simulink model "ExampleBlindSpot"  (Simulink 9.2)
settings: Solver=FixedStepDiscrete  StartTime=0.0  StopTime=Inf  FixedStep=0.001  RelTol=1e-3  EnableMultiTasking=on
libraries: simulink x30, rFproPhysicsLib x6, simulink_extras x3
settings Model: Creator=SeanK  LastModifiedBy=SeanKavanagh
settings DataIOCC: SignalLoggingSaveFormat=Dataset
settings DebuggingCC: SolverPrmCheckMsg=warning  FcnCallInpInsideContextMsg=error  StateNameClashWarn=none
settings RTWCC: SystemTargetFile=rfpro.tlc  MakeCommand="make_rtw OPTS=\"-DRUN_PHYSICS\""  TemplateMakefile=rfpro.tmf  Description=rFpro Target (Run Physics)  TargetLang=C++
settings STFCustomTargetCC: ModelReferenceCompliant=off  GeneratePreprocessorConditionals=Disable all  CombineOutputUpdateFcns=on  MatFileLogging=on  CPPClassGenCompliant=on  GRTInterface=off  SystemTargetFile=rfpro.tlc
settings GRTTargetCC: ModelReferenceCompliant=off  ParMdlRefBuildCompliant=off  CompOptLevelCompliant=off  ConcurrentExecutionCompliant=off  CombineOutputUpdateFcns=on  GRTInterface=off  UseToolchainInfoCompliant=off

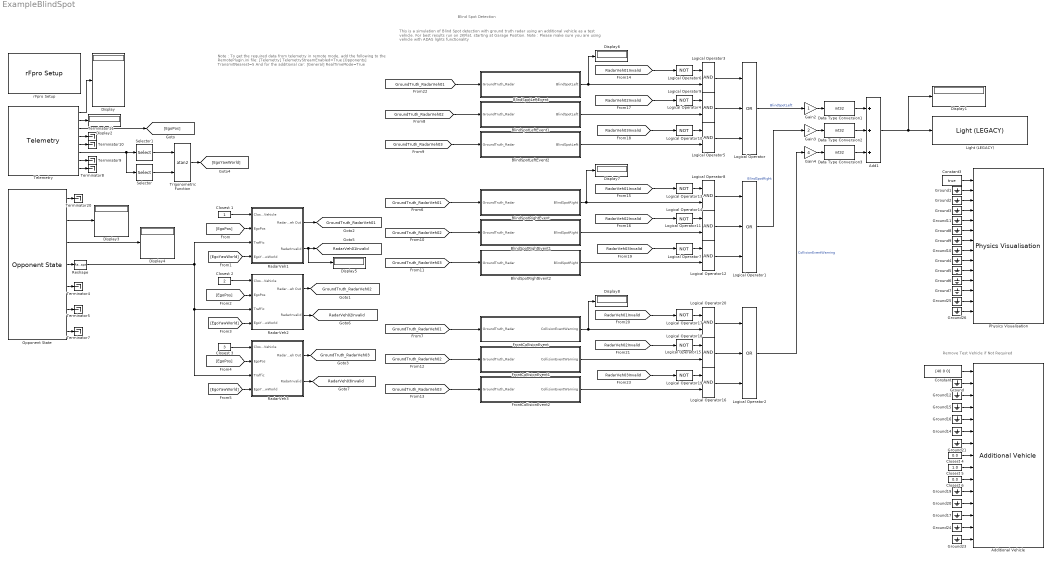
== system ExampleBlindSpot ==
  note: This is a simulation of Blind Spot detection with ground truth radar using an additional vehicle as a test vehicle.
      | For best results run on 2KFlat, starting at Garage Position.
      | Note : Please make sure you are using vehicle with ADAS lights functionality
  note: Remove Test Vehicle if Not Required
  note: Blind Spot Detection
  note: Note : To get the required data from telemetry in remote mode,
      | add the following to the RemotePlugin.ini file:
      |
      | [Telemetry]
      | TelemetryStreamEnabled=True
      |
      | [Opponents]
      | TransmitNearest=5
      |
      | And for the additional car:
      |
      | [General]
      | RealTimeMode=True
  Add1 : Sum  Inputs=+++
  Additional Vehicle : rFproPhysicsLib/Additional Vehicle  VEH_FILE='Hatchback_AWD_Red'  DRIVER_NAME=''  UPGRADE_PACK=0  SKIN=''  HELMET=''  COLLIDABLE=off  TRANSPARENT_PROXIMITY=0  MANUAL_TRANSPARENCY=0  HEIGHT_VALID=off  ORI_VALID=off  HEADING_VALID=off  VEL_VALID=off  ROT_VALID=off  GEAR_VALID=off  RPM_VALID=off  INPUTS_VALID=on  BRAKE_LIGHT_VALID=off  HEADLIGHT_VALID=off  WHEEL_ROTATIONS_VALID=off  WHEEL_BRAKE_TEMPS_VALID=off  WHEEL_HEIGHTS_VALID=off  period=-1  offset=0  useReverseByteOrder=on  rFpro__platform=Remote Model - Default
  BlindSpotLeftEvent : Subsystem
  BlindSpotLeftEvent1 : Subsystem
  BlindSpotLeftEvent2 : Subsystem
  BlindSpotRightEvent : Subsystem
  BlindSpotRightEvent1 : Subsystem
  BlindSpotRightEvent2 : Subsystem
  Closest 1 : Constant
  Closest 2 : Constant  Value=2
  Closest 3 : Constant  Value=3
  Closest 4 : Constant  Value=0.0
  Closest 5 : Constant  Value=1.0
  Closest 6 : Constant  Value=0.0
  Constant : Constant  Value=[40 0 0]
  Constant3 : Constant  Value=true
  Data Type Conversion1 : DataTypeConversion  OutDataTypeStr=int32
  Data Type Conversion2 : DataTypeConversion  OutDataTypeStr=int32
  Data Type Conversion3 : DataTypeConversion  OutDataTypeStr=int32
  Display{,1..8} (9 alike) : Display
  FrontCollisionEvent : Subsystem
  FrontCollisionEvent1 : Subsystem
  FrontCollisionEvent2 : Subsystem
  Gain2 : Gain
  Gain3 : Gain  Gain=2
  Gain4 : Gain  Gain=4
  Ground{,1..12,14..17,19..21,23..26} (24 alike) : Ground
  Light (LEGACY) : rFproPhysicsLib/Legacy Blocks/Light (LEGACY)  light_name='LIGHTSADAS'  exact_match=off  on_vehicle=on  useReverseByteOrder=off  rFpro__platform=Remote Model - Default
  Logical Operator : Logic  Operator=OR  Inputs=3  AllPortsSameDT=off  OutDataTypeStr=boolean
  Logical Operator1 : Logic  Operator=OR  Inputs=3  AllPortsSameDT=off  OutDataTypeStr=boolean
  Logical Operator{6..7,9..10,13..14,17..19} (9 alike) : Logic  Operator=NOT  AllPortsSameDT=off  OutDataTypeStr=boolean
  Logical Operator{3..5,8,11..12,15..16,20} (9 alike) : Logic  AllPortsSameDT=off  OutDataTypeStr=boolean
  Logical Operator2 : Logic  Operator=OR  Inputs=3  AllPortsSameDT=off  OutDataTypeStr=boolean
  Opponent State : rFproPhysicsLib/Opponent State  max_SL_opponents=3  flattenOutput=on
  Physics Visualisation : rFproPhysicsLib/Physics Visualisation  PAR_SKIP_INTERNAL_PHYSICS=off  PAR_ACCEL_VALID=off  PAR_ROT_ACCEL_VALID=off  PAR_GEAR_VALID=off  PAR_RPM_VALID=off  PAR_INPUTS_VALID=on  PAR_STEER_TORQUE_VALID=off  PAR_HEADLIGHTS_ON_VALID=off  PAR_WHEEL_POS_VALID=off  PAR_WHEEL_ORI_VALID=off  PAR_TYRE_PARAMS_VALID=off  PAR_WHEEL_ROTATION_VALID=off  PAR_WHEEL_BRAKE_TEMP_VALID=off  PAR_WHEEL_TREAD_TEMP_VALID=off  PAR_WHEEL_AIR_TEMP_VALID=off  period=-1  offset=0  useReverseByteOrder=on  rFpro__platform=Remote Model - Default
  RadarVeh1 : Subsystem
  RadarVeh2 : Subsystem
  RadarVeh3 : Subsystem
  Reshape : Reshape  OutputDimensionality=Customize  OutputDimensions=[3,3]
  Selector : Selector  NumberOfDimensions=2  InputPortWidth=3  IndexOptions=Index vector (dialog),Index vector (dialog)  Indices=1,1  OutputSizes=1,1
  Selector1 : Selector  NumberOfDimensions=2  InputPortWidth=3  IndexOptions=Index vector (dialog),Index vector (dialog)  Indices=1,2  OutputSizes=1,1
  Telemetry : rFproPhysicsLib/Telemetry
  Terminator{4..5,7..11,20} (8 alike) : Terminator
  Trigonometric Function : Trigonometry  Operator=atan2
  rFpro Setup : rFproPhysicsLib/rFpro Setup  platform=Remote Model - Default  stopOnSessionEnd=on  usePseudoRealtime=on  syncToRF=on  useReverseByteOrder=off  useRfTime=on  minIterations=4  maxIterations=1000  ipReceiveAddress='127.0.0.1'  ipReceivePort=11054  receiveSampleTime=-1  ipTransmitAddress='127.0.0.1'  ipTransmitPort=11052  transmitSampleTime=0.001  pluginType=RUN_PHYSICS  sysTarget=xpctarget.tlc  templateMakeFile=xpc_default_tmf  makeCommand=make_rtw  buildDesc=xPC target
  tag scope: GroundTruth_RadarVeh01=global, GroundTruth_RadarVeh02=global, GroundTruth_RadarVeh03=global, RadarVeh01Invalid=global, RadarVeh02Invalid=global, RadarVeh03Invalid=global
  wires:
  Constant3/1 -> Physics Visualisation/1
  Ground8/1 -> Physics Visualisation/6
  Ground9/1 -> Physics Visualisation/7
  Ground10/1 -> Physics Visualisation/8
  Ground11/1 -> Physics Visualisation/5
  Ground1/1 -> Physics Visualisation/2
  Ground2/1 -> Physics Visualisation/3
  Ground3/1 -> Physics Visualisation/4
  Opponent State/2 -> Display3/1
  Opponent State/5 -> Terminator4/1
  Opponent State/6 -> Terminator5/1
  Closest 1/1 -> RadarVeh1/1(Closest Vehicle)
  Telemetry/3 -> [EgoPos]
  [EgoYawWorld] -> RadarVeh1/4(EgoYawWorld)
  [EgoPos] -> RadarVeh1/2(EgoPos)
  [EgoPos] -> RadarVeh2/2(EgoPos)
  [EgoYawWorld] -> RadarVeh2/4(EgoYawWorld)
  Closest 2/1 -> RadarVeh2/1(Closest Vehicle)
  Closest 3/1 -> RadarVeh3/1(Closest Vehicle)
  [EgoYawWorld] -> RadarVeh3/4(EgoYawWorld)
  [EgoPos] -> RadarVeh3/2(EgoPos)
  RadarVeh1/1(RadarVeh Out) -> [GroundTruth_RadarVeh01]
  RadarVeh2/1(RadarVeh Out) -> [GroundTruth_RadarVeh02]
  RadarVeh3/1(RadarVeh Out) -> [GroundTruth_RadarVeh03]
  Logical Operator2/1 -> Gain4/1  "CollisionEventWarning"
  Logical Operator/1 -> Gain2/1  "BlindSpotLeft"
  Logical Operator1/1 -> Gain3/1  "BlindSpotRight"
  [GroundTruth_RadarVeh03] -> FrontCollisionEvent2/1(GroundTruth_Radar)
  [GroundTruth_RadarVeh02] -> FrontCollisionEvent1/1(GroundTruth_Radar)
  [GroundTruth_RadarVeh03] -> BlindSpotRightEvent2/1(GroundTruth_Radar)
  [GroundTruth_RadarVeh02] -> BlindSpotRightEvent1/1(GroundTruth_Radar)
  BlindSpotLeftEvent2/1(BlindSpotLeft) -> Logical Operator5/2
  [GroundTruth_RadarVeh03] -> BlindSpotLeftEvent2/1(GroundTruth_Radar)
  [GroundTruth_RadarVeh02] -> BlindSpotLeftEvent1/1(GroundTruth_Radar)
  BlindSpotLeftEvent1/1(BlindSpotLeft) -> Logical Operator4/2
  [GroundTruth_RadarVeh01] -> FrontCollisionEvent/1(GroundTruth_Radar)
  [GroundTruth_RadarVeh01] -> BlindSpotRightEvent/1(GroundTruth_Radar)
  BlindSpotLeftEvent/1(BlindSpotLeft) -> Display6/1, Logical Operator3/2
  [GroundTruth_RadarVeh01] -> BlindSpotLeftEvent/1(GroundTruth_Radar)
  Gain4/1 -> Data Type Conversion3/1
  Add1/1 -> Light (LEGACY)/1, Display1/1
  Gain3/1 -> Data Type Conversion2/1
  Data Type Conversion1/1 -> Add1/1
  Data Type Conversion3/1 -> Add1/3
  Data Type Conversion2/1 -> Add1/2
  Gain2/1 -> Data Type Conversion1/1
  Trigonometric Function/1 -> [EgoYawWorld]
  Constant/1 -> Additional Vehicle/1
  Ground/1 -> Additional Vehicle/2
  Ground19/1 -> Additional Vehicle/11
  Ground16/1 -> Additional Vehicle/5
  Ground15/1 -> Additional Vehicle/4
  Ground12/1 -> Additional Vehicle/3
  Ground20/1 -> Additional Vehicle/12
  Ground17/1 -> Additional Vehicle/13
  Ground14/1 -> Additional Vehicle/6
  Ground21/1 -> Additional Vehicle/7
  Ground24/1 -> Additional Vehicle/14
  Ground23/1 -> Additional Vehicle/15
  Telemetry/6 -> Selector/1, Selector1/1
  Selector1/1 -> Trigonometric Function/1
  Selector/1 -> Trigonometric Function/2
  RadarVeh1/2(RadarInvalid) -> Display5/1, [RadarVeh01Invalid]
  RadarVeh2/2(RadarInvalid) -> [RadarVeh02Invalid]
  RadarVeh3/2(RadarInvalid) -> [RadarVeh03Invalid]
  [RadarVeh01Invalid] -> Logical Operator6/1
  Logical Operator6/1 -> Logical Operator3/1
  Logical Operator3/1 -> Logical Operator/1
  Logical Operator4/1 -> Logical Operator/2
  Logical Operator5/1 -> Logical Operator/3
  Logical Operator9/1 -> Logical Operator4/1
  [RadarVeh02Invalid] -> Logical Operator9/1
  [RadarVeh03Invalid] -> Logical Operator10/1
  Logical Operator10/1 -> Logical Operator5/1
  Logical Operator7/1 -> Logical Operator12/1
  [RadarVeh03Invalid] -> Logical Operator7/1
  [RadarVeh02Invalid] -> Logical Operator14/1
  Logical Operator14/1 -> Logical Operator11/1
  Logical Operator12/1 -> Logical Operator1/3
  Logical Operator11/1 -> Logical Operator1/2
  Logical Operator8/1 -> Logical Operator1/1
  Logical Operator13/1 -> Logical Operator8/1
  [RadarVeh01Invalid] -> Logical Operator13/1
  BlindSpotRightEvent/1(BlindSpotRight) -> Display7/1, Logical Operator8/2
  BlindSpotRightEvent1/1(BlindSpotRight) -> Logical Operator11/2
  BlindSpotRightEvent2/1(BlindSpotRight) -> Logical Operator12/2
  FrontCollisionEvent2/1(CollisionEventWarning) -> Logical Operator16/2
  FrontCollisionEvent1/1(CollisionEventWarning) -> Logical Operator15/2
  FrontCollisionEvent/1(CollisionEventWarning) -> Display8/1, Logical Operator20/2
  [RadarVeh01Invalid] -> Logical Operator17/1
  Logical Operator17/1 -> Logical Operator20/1
  Logical Operator20/1 -> Logical Operator2/1
  Logical Operator15/1 -> Logical Operator2/2
  Logical Operator16/1 -> Logical Operator2/3
  Logical Operator18/1 -> Logical Operator15/1
  [RadarVeh02Invalid] -> Logical Operator18/1
  [RadarVeh03Invalid] -> Logical Operator19/1
  Logical Operator19/1 -> Logical Operator16/1
  Opponent State/1 -> Terminator20/1
  Ground4/1 -> Physics Visualisation/9
  Ground5/1 -> Physics Visualisation/10
  Ground6/1 -> Physics Visualisation/11
  Ground7/1 -> Physics Visualisation/12
  Ground26/1 -> Physics Visualisation/14
  Ground25/1 -> Physics Visualisation/13
  Opponent State/7 -> Terminator7/1
  Opponent State/4 -> Reshape/1
  Telemetry/1 -> Display/1
  Telemetry/2 -> Display2/1
  Telemetry/4 -> Terminator11/1
  Telemetry/5 -> Terminator10/1
  Telemetry/7 -> Terminator9/1
  Telemetry/8 -> Terminator8/1
  Opponent State/3 -> Display4/1
  Reshape/1 -> RadarVeh1/3(Traffic), RadarVeh3/3(Traffic), RadarVeh2/3(Traffic)
  Closest 4/1 -> Additional Vehicle/8
  Closest 5/1 -> Additional Vehicle/9
  Closest 6/1 -> Additional Vehicle/10

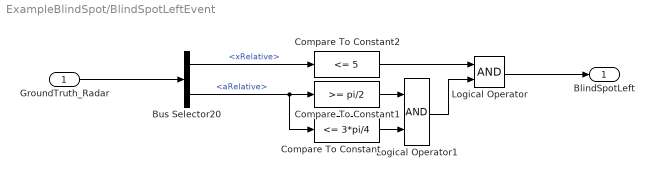
== system ExampleBlindSpot/BlindSpotLeftEvent ==
  GroundTruth_Radar : Inport
  Bus Selector20 : BusSelector  OutputSignals=xRelative,aRelative
  Compare To Constant : simulink/Logic and Bit Operations/Compare To Constant  relop=<=  const=3*pi/4  OutDataTypeStr=boolean
  Compare To Constant1 : simulink/Logic and Bit Operations/Compare To Constant  relop=>=  const=pi/2  OutDataTypeStr=boolean
  Compare To Constant2 : simulink/Logic and Bit Operations/Compare To Constant  relop=<=  const=5  OutDataTypeStr=boolean
  Logical Operator : Logic  AllPortsSameDT=off  OutDataTypeStr=boolean
  Logical Operator1 : Logic  AllPortsSameDT=off  OutDataTypeStr=boolean
  BlindSpotLeft : Outport
  wires:
  Logical Operator/1 -> BlindSpotLeft/1
  Compare To Constant2/1 -> Logical Operator/1
  Logical Operator1/1 -> Logical Operator/2
  Bus Selector20/1 -> Compare To Constant2/1  "<xRelative>"
  GroundTruth_Radar/1 -> Bus Selector20/1
  Compare To Constant1/1 -> Logical Operator1/1
  Bus Selector20/2 -> Compare To Constant/1, Compare To Constant1/1  "<aRelative>"
  Compare To Constant/1 -> Logical Operator1/2

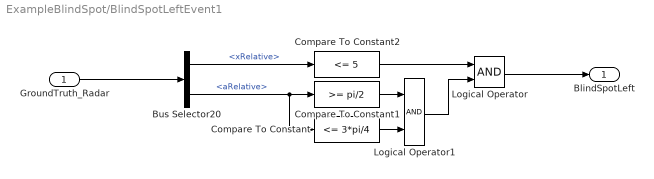
== system ExampleBlindSpot/BlindSpotLeftEvent1 ==
  GroundTruth_Radar : Inport
  Bus Selector20 : BusSelector  OutputSignals=xRelative,aRelative
  Compare To Constant : simulink/Logic and Bit Operations/Compare To Constant  relop=<=  const=3*pi/4  OutDataTypeStr=boolean
  Compare To Constant1 : simulink/Logic and Bit Operations/Compare To Constant  relop=>=  const=pi/2  OutDataTypeStr=boolean
  Compare To Constant2 : simulink/Logic and Bit Operations/Compare To Constant  relop=<=  const=5  OutDataTypeStr=boolean
  Logical Operator : Logic  AllPortsSameDT=off  OutDataTypeStr=boolean
  Logical Operator1 : Logic  AllPortsSameDT=off  OutDataTypeStr=boolean
  BlindSpotLeft : Outport
  wires:
  Logical Operator/1 -> BlindSpotLeft/1
  Compare To Constant2/1 -> Logical Operator/1
  Logical Operator1/1 -> Logical Operator/2
  Bus Selector20/1 -> Compare To Constant2/1  "<xRelative>"
  GroundTruth_Radar/1 -> Bus Selector20/1
  Compare To Constant1/1 -> Logical Operator1/1
  Bus Selector20/2 -> Compare To Constant/1, Compare To Constant1/1  "<aRelative>"
  Compare To Constant/1 -> Logical Operator1/2

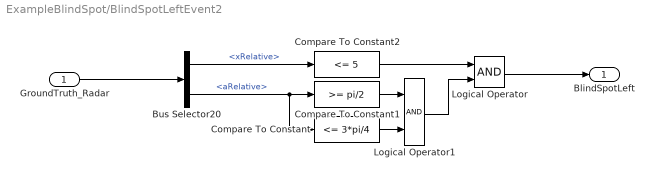
== system ExampleBlindSpot/BlindSpotLeftEvent2 ==
  GroundTruth_Radar : Inport
  Bus Selector20 : BusSelector  OutputSignals=xRelative,aRelative
  Compare To Constant : simulink/Logic and Bit Operations/Compare To Constant  relop=<=  const=3*pi/4  OutDataTypeStr=boolean
  Compare To Constant1 : simulink/Logic and Bit Operations/Compare To Constant  relop=>=  const=pi/2  OutDataTypeStr=boolean
  Compare To Constant2 : simulink/Logic and Bit Operations/Compare To Constant  relop=<=  const=5  OutDataTypeStr=boolean
  Logical Operator : Logic  AllPortsSameDT=off  OutDataTypeStr=boolean
  Logical Operator1 : Logic  AllPortsSameDT=off  OutDataTypeStr=boolean
  BlindSpotLeft : Outport
  wires:
  Logical Operator/1 -> BlindSpotLeft/1
  Compare To Constant2/1 -> Logical Operator/1
  Logical Operator1/1 -> Logical Operator/2
  Bus Selector20/1 -> Compare To Constant2/1  "<xRelative>"
  GroundTruth_Radar/1 -> Bus Selector20/1
  Compare To Constant1/1 -> Logical Operator1/1
  Bus Selector20/2 -> Compare To Constant/1, Compare To Constant1/1  "<aRelative>"
  Compare To Constant/1 -> Logical Operator1/2

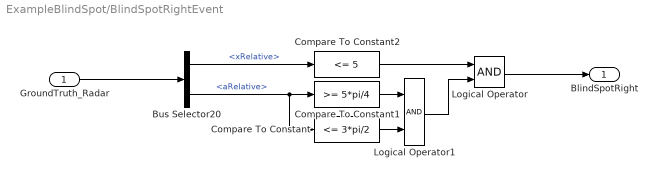
== system ExampleBlindSpot/BlindSpotRightEvent ==
  GroundTruth_Radar : Inport
  Bus Selector20 : BusSelector  OutputSignals=xRelative,aRelative
  Compare To Constant : simulink/Logic and Bit Operations/Compare To Constant  relop=<=  const=3*pi/2  OutDataTypeStr=boolean
  Compare To Constant1 : simulink/Logic and Bit Operations/Compare To Constant  relop=>=  const=5*pi/4  OutDataTypeStr=boolean
  Compare To Constant2 : simulink/Logic and Bit Operations/Compare To Constant  relop=<=  const=5  OutDataTypeStr=boolean
  Logical Operator : Logic  AllPortsSameDT=off  OutDataTypeStr=boolean
  Logical Operator1 : Logic  AllPortsSameDT=off  OutDataTypeStr=boolean
  BlindSpotRight : Outport
  wires:
  Compare To Constant/1 -> Logical Operator1/2
  Bus Selector20/2 -> Compare To Constant/1, Compare To Constant1/1  "<aRelative>"
  Compare To Constant1/1 -> Logical Operator1/1
  GroundTruth_Radar/1 -> Bus Selector20/1
  Bus Selector20/1 -> Compare To Constant2/1  "<xRelative>"
  Logical Operator1/1 -> Logical Operator/2
  Compare To Constant2/1 -> Logical Operator/1
  Logical Operator/1 -> BlindSpotRight/1

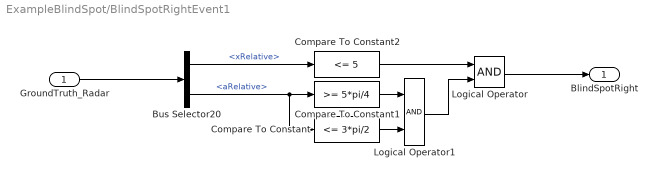
== system ExampleBlindSpot/BlindSpotRightEvent1 ==
  GroundTruth_Radar : Inport
  Bus Selector20 : BusSelector  OutputSignals=xRelative,aRelative
  Compare To Constant : simulink/Logic and Bit Operations/Compare To Constant  relop=<=  const=3*pi/2  OutDataTypeStr=boolean
  Compare To Constant1 : simulink/Logic and Bit Operations/Compare To Constant  relop=>=  const=5*pi/4  OutDataTypeStr=boolean
  Compare To Constant2 : simulink/Logic and Bit Operations/Compare To Constant  relop=<=  const=5  OutDataTypeStr=boolean
  Logical Operator : Logic  AllPortsSameDT=off  OutDataTypeStr=boolean
  Logical Operator1 : Logic  AllPortsSameDT=off  OutDataTypeStr=boolean
  BlindSpotRight : Outport
  wires:
  Compare To Constant/1 -> Logical Operator1/2
  Bus Selector20/2 -> Compare To Constant/1, Compare To Constant1/1  "<aRelative>"
  Compare To Constant1/1 -> Logical Operator1/1
  GroundTruth_Radar/1 -> Bus Selector20/1
  Bus Selector20/1 -> Compare To Constant2/1  "<xRelative>"
  Logical Operator1/1 -> Logical Operator/2
  Compare To Constant2/1 -> Logical Operator/1
  Logical Operator/1 -> BlindSpotRight/1

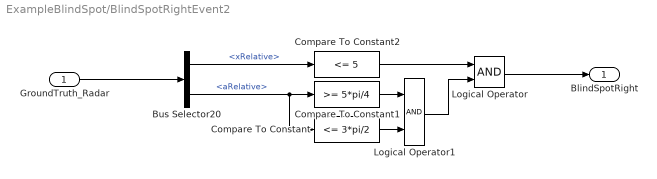
== system ExampleBlindSpot/BlindSpotRightEvent2 ==
  GroundTruth_Radar : Inport
  Bus Selector20 : BusSelector  OutputSignals=xRelative,aRelative
  Compare To Constant : simulink/Logic and Bit Operations/Compare To Constant  relop=<=  const=3*pi/2  OutDataTypeStr=boolean
  Compare To Constant1 : simulink/Logic and Bit Operations/Compare To Constant  relop=>=  const=5*pi/4  OutDataTypeStr=boolean
  Compare To Constant2 : simulink/Logic and Bit Operations/Compare To Constant  relop=<=  const=5  OutDataTypeStr=boolean
  Logical Operator : Logic  AllPortsSameDT=off  OutDataTypeStr=boolean
  Logical Operator1 : Logic  AllPortsSameDT=off  OutDataTypeStr=boolean
  BlindSpotRight : Outport
  wires:
  Compare To Constant/1 -> Logical Operator1/2
  Bus Selector20/2 -> Compare To Constant/1, Compare To Constant1/1  "<aRelative>"
  Compare To Constant1/1 -> Logical Operator1/1
  GroundTruth_Radar/1 -> Bus Selector20/1
  Bus Selector20/1 -> Compare To Constant2/1  "<xRelative>"
  Logical Operator1/1 -> Logical Operator/2
  Compare To Constant2/1 -> Logical Operator/1
  Logical Operator/1 -> BlindSpotRight/1

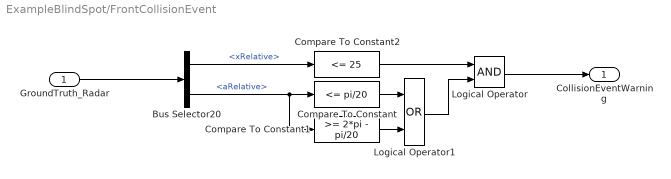
== system ExampleBlindSpot/FrontCollisionEvent ==
  GroundTruth_Radar : Inport
  Bus Selector20 : BusSelector  OutputSignals=xRelative,aRelative
  Compare To Constant : simulink/Logic and Bit Operations/Compare To Constant  relop=<=  const=pi/20  OutDataTypeStr=boolean
  Compare To Constant1 : simulink/Logic and Bit Operations/Compare To Constant  relop=>=  const=2*pi - pi/20  OutDataTypeStr=boolean
  Compare To Constant2 : simulink/Logic and Bit Operations/Compare To Constant  relop=<=  const=25  OutDataTypeStr=boolean
  Logical Operator : Logic  AllPortsSameDT=off  OutDataTypeStr=boolean
  Logical Operator1 : Logic  Operator=OR  AllPortsSameDT=off  OutDataTypeStr=boolean
  CollisionEventWarning : Outport
  wires:
  Compare To Constant/1 -> Logical Operator1/1
  Bus Selector20/2 -> Compare To Constant1/1, Compare To Constant/1  "<aRelative>"
  Compare To Constant1/1 -> Logical Operator1/2
  GroundTruth_Radar/1 -> Bus Selector20/1
  Bus Selector20/1 -> Compare To Constant2/1  "<xRelative>"
  Logical Operator1/1 -> Logical Operator/2
  Compare To Constant2/1 -> Logical Operator/1
  Logical Operator/1 -> CollisionEventWarning/1

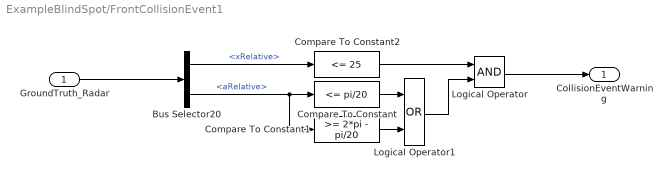
== system ExampleBlindSpot/FrontCollisionEvent1 ==
  GroundTruth_Radar : Inport
  Bus Selector20 : BusSelector  OutputSignals=xRelative,aRelative
  Compare To Constant : simulink/Logic and Bit Operations/Compare To Constant  relop=<=  const=pi/20  OutDataTypeStr=boolean
  Compare To Constant1 : simulink/Logic and Bit Operations/Compare To Constant  relop=>=  const=2*pi - pi/20  OutDataTypeStr=boolean
  Compare To Constant2 : simulink/Logic and Bit Operations/Compare To Constant  relop=<=  const=25  OutDataTypeStr=boolean
  Logical Operator : Logic  AllPortsSameDT=off  OutDataTypeStr=boolean
  Logical Operator1 : Logic  Operator=OR  AllPortsSameDT=off  OutDataTypeStr=boolean
  CollisionEventWarning : Outport
  wires:
  Compare To Constant/1 -> Logical Operator1/1
  Bus Selector20/2 -> Compare To Constant1/1, Compare To Constant/1  "<aRelative>"
  Compare To Constant1/1 -> Logical Operator1/2
  GroundTruth_Radar/1 -> Bus Selector20/1
  Bus Selector20/1 -> Compare To Constant2/1  "<xRelative>"
  Logical Operator1/1 -> Logical Operator/2
  Compare To Constant2/1 -> Logical Operator/1
  Logical Operator/1 -> CollisionEventWarning/1

== system ExampleBlindSpot/FrontCollisionEvent2 ==
  GroundTruth_Radar : Inport
  Bus Selector20 : BusSelector  OutputSignals=xRelative,aRelative
  Compare To Constant : simulink/Logic and Bit Operations/Compare To Constant  relop=<=  const=pi/20  OutDataTypeStr=boolean
  Compare To Constant1 : simulink/Logic and Bit Operations/Compare To Constant  relop=>=  const=2*pi - pi/20  OutDataTypeStr=boolean
  Compare To Constant2 : simulink/Logic and Bit Operations/Compare To Constant  relop=<=  const=25  OutDataTypeStr=boolean
  Logical Operator : Logic  AllPortsSameDT=off  OutDataTypeStr=boolean
  Logical Operator1 : Logic  Operator=OR  AllPortsSameDT=off  OutDataTypeStr=boolean
  CollisionEventWarning : Outport
  wires:
  Compare To Constant/1 -> Logical Operator1/1
  Bus Selector20/2 -> Compare To Constant1/1, Compare To Constant/1  "<aRelative>"
  Compare To Constant1/1 -> Logical Operator1/2
  GroundTruth_Radar/1 -> Bus Selector20/1
  Bus Selector20/1 -> Compare To Constant2/1  "<xRelative>"
  Logical Operator1/1 -> Logical Operator/2
  Compare To Constant2/1 -> Logical Operator/1
  Logical Operator/1 -> CollisionEventWarning/1

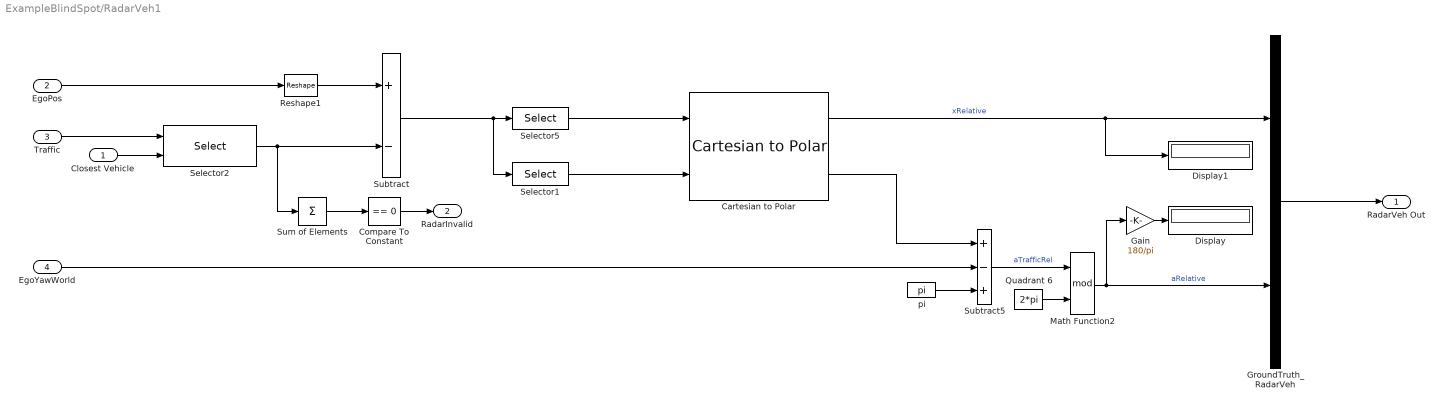
== system ExampleBlindSpot/RadarVeh1 ==
  Closest Vehicle : Inport
  EgoPos : Inport  Port=2
  Traffic : Inport  Port=3
  EgoYawWorld : Inport  Port=4
  Cartesian to Polar : simulink_extras/Transformations/Cartesian to Polar
      settings: SourceProductName=Simulink
  Compare To Constant : simulink/Logic and Bit Operations/Compare To Constant  relop===  const=0  OutDataTypeStr=boolean
  Display : Display
  Display1 : Display
  Gain : Gain  Gain=180/pi
  GroundTruth_RadarVeh : BusCreator  Inputs=2
  Math Function2 : Math  Operator=mod  SaturateOnIntegerOverflow=on
  Quadrant 6 : Constant  Value=2*pi
  Reshape1 : Reshape  OutputDimensionality=Column vector (2-D)
  Selector1 : Selector  InputPortWidth=3  IndexOptions=Index vector (dialog)  Indices=2  OutputSizes=1
  Selector2 : Selector  NumberOfDimensions=2  InputPortWidth=3  IndexOptions=Select all,Index vector (port)  Indices=[1 2 3],[1 2 3]  OutputSizes=1,1
  Selector5 : Selector  InputPortWidth=3  IndexOptions=Index vector (dialog)  Indices=1  OutputSizes=1
  Subtract : Sum  Inputs=+-
  Subtract5 : Sum  Inputs=+-+
  Sum of Elements : Sum  Inputs=+
  pi : Constant  Value=pi
  RadarVeh Out : Outport
  RadarInvalid : Outport  Port=2
  wires:
  Math Function2/1 -> GroundTruth_RadarVeh/2, Gain/1  "aRelative"
  EgoYawWorld/1 -> Subtract5/2
  Cartesian to Polar/1 -> Display1/1, GroundTruth_RadarVeh/1  "xRelative"
  Reshape1/1 -> Subtract/1
  Closest Vehicle/1 -> Selector2/2
  EgoPos/1 -> Reshape1/1
  Traffic/1 -> Selector2/1
  Selector2/1 -> Sum of Elements/1, Subtract/2
  GroundTruth_RadarVeh/1 -> RadarVeh Out/1
  pi/1 -> Subtract5/3
  Quadrant 6/1 -> Math Function2/2
  Subtract5/1 -> Math Function2/1  "aTrafficRel"
  Cartesian to Polar/2 -> Subtract5/1
  Selector5/1 -> Cartesian to Polar/1
  Selector1/1 -> Cartesian to Polar/2
  Subtract/1 -> Selector1/1, Selector5/1
  Compare To Constant/1 -> RadarInvalid/1
  Sum of Elements/1 -> Compare To Constant/1
  Gain/1 -> Display/1

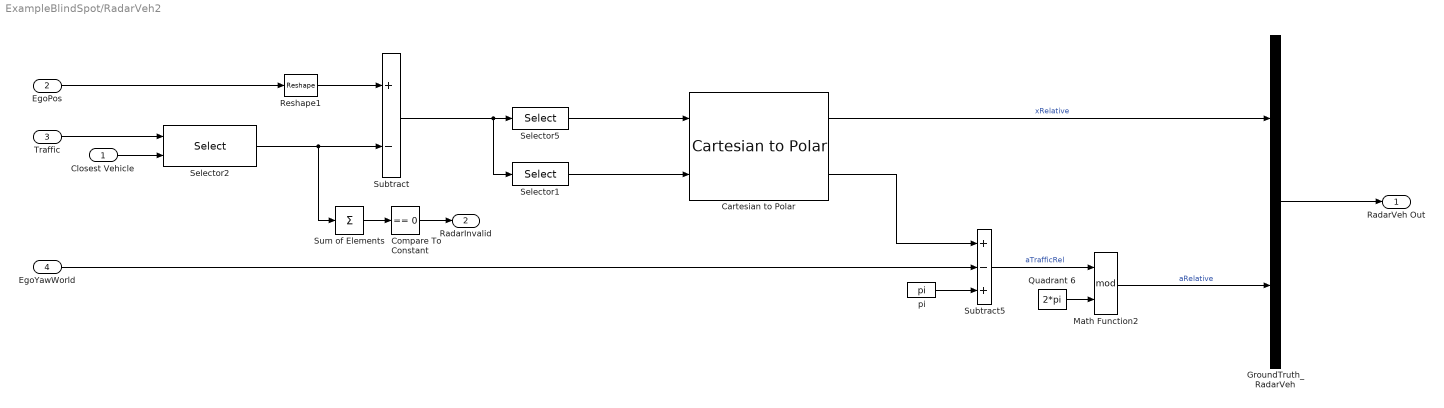
== system ExampleBlindSpot/RadarVeh2 ==
  Closest Vehicle : Inport
  EgoPos : Inport  Port=2
  Traffic : Inport  Port=3
  EgoYawWorld : Inport  Port=4
  Cartesian to Polar : simulink_extras/Transformations/Cartesian to Polar
      settings: SourceProductName=Simulink
  Compare To Constant : simulink/Logic and Bit Operations/Compare To Constant  relop===  const=0  OutDataTypeStr=boolean
  GroundTruth_RadarVeh : BusCreator  Inputs=2
  Math Function2 : Math  Operator=mod  SaturateOnIntegerOverflow=on
  Quadrant 6 : Constant  Value=2*pi
  Reshape1 : Reshape  OutputDimensionality=Column vector (2-D)
  Selector1 : Selector  InputPortWidth=3  IndexOptions=Index vector (dialog)  Indices=2  OutputSizes=1
  Selector2 : Selector  NumberOfDimensions=2  InputPortWidth=3  IndexOptions=Index vector (dialog),Index vector (port)  Indices=[1 2 3],[1 2 3]  OutputSizes=1,1
  Selector5 : Selector  InputPortWidth=3  IndexOptions=Index vector (dialog)  Indices=1  OutputSizes=1
  Subtract : Sum  Inputs=+-
  Subtract5 : Sum  Inputs=+-+
  Sum of Elements : Sum  Inputs=+
  pi : Constant  Value=pi
  RadarVeh Out : Outport
  RadarInvalid : Outport  Port=2
  wires:
  Subtract/1 -> Selector5/1, Selector1/1
  Selector1/1 -> Cartesian to Polar/2
  Selector5/1 -> Cartesian to Polar/1
  Cartesian to Polar/2 -> Subtract5/1
  Subtract5/1 -> Math Function2/1  "aTrafficRel"
  Quadrant 6/1 -> Math Function2/2
  pi/1 -> Subtract5/3
  GroundTruth_RadarVeh/1 -> RadarVeh Out/1
  Traffic/1 -> Selector2/1
  EgoPos/1 -> Reshape1/1
  Closest Vehicle/1 -> Selector2/2
  Reshape1/1 -> Subtract/1
  Cartesian to Polar/1 -> GroundTruth_RadarVeh/1  "xRelative"
  EgoYawWorld/1 -> Subtract5/2
  Math Function2/1 -> GroundTruth_RadarVeh/2  "aRelative"
  Selector2/1 -> Sum of Elements/1, Subtract/2
  Compare To Constant/1 -> RadarInvalid/1
  Sum of Elements/1 -> Compare To Constant/1

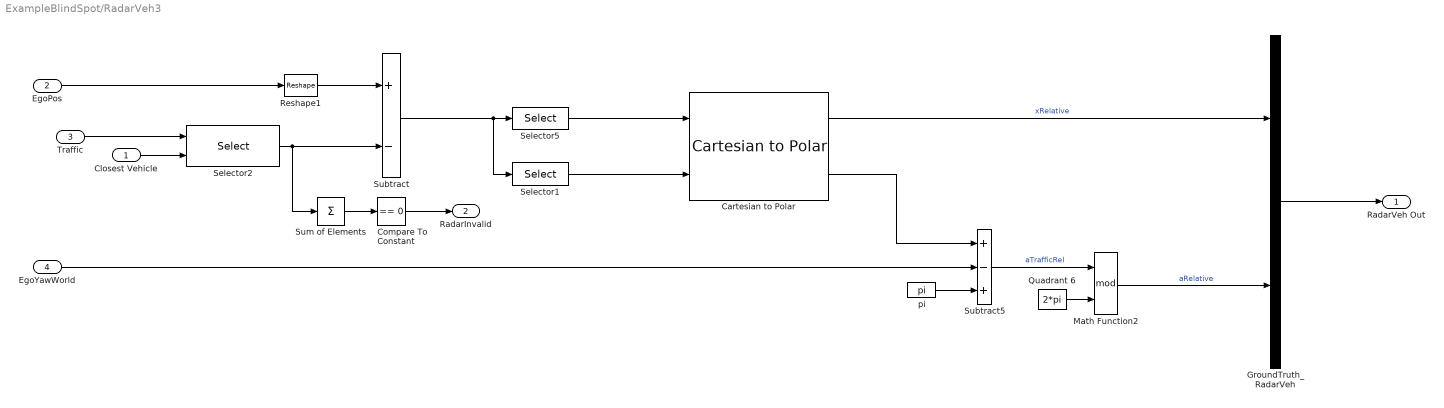
== system ExampleBlindSpot/RadarVeh3 ==
  Closest Vehicle : Inport
  EgoPos : Inport  Port=2
  Traffic : Inport  Port=3
  EgoYawWorld : Inport  Port=4
  Cartesian to Polar : simulink_extras/Transformations/Cartesian to Polar
      settings: SourceProductName=Simulink
  Compare To Constant : simulink/Logic and Bit Operations/Compare To Constant  relop===  const=0  OutDataTypeStr=boolean
  GroundTruth_RadarVeh : BusCreator  Inputs=2
  Math Function2 : Math  Operator=mod  SaturateOnIntegerOverflow=on
  Quadrant 6 : Constant  Value=2*pi
  Reshape1 : Reshape  OutputDimensionality=Column vector (2-D)
  Selector1 : Selector  InputPortWidth=3  IndexOptions=Index vector (dialog)  Indices=2  OutputSizes=1
  Selector2 : Selector  NumberOfDimensions=2  InputPortWidth=3  IndexOptions=Index vector (dialog),Index vector (port)  Indices=[1 2 3],[1 2 3]  OutputSizes=1,1
  Selector5 : Selector  InputPortWidth=3  IndexOptions=Index vector (dialog)  Indices=1  OutputSizes=1
  Subtract : Sum  Inputs=+-
  Subtract5 : Sum  Inputs=+-+
  Sum of Elements : Sum  Inputs=+
  pi : Constant  Value=pi
  RadarVeh Out : Outport
  RadarInvalid : Outport  Port=2
  wires:
  Math Function2/1 -> GroundTruth_RadarVeh/2  "aRelative"
  EgoYawWorld/1 -> Subtract5/2
  Cartesian to Polar/1 -> GroundTruth_RadarVeh/1  "xRelative"
  Reshape1/1 -> Subtract/1
  Closest Vehicle/1 -> Selector2/2
  EgoPos/1 -> Reshape1/1
  Traffic/1 -> Selector2/1
  GroundTruth_RadarVeh/1 -> RadarVeh Out/1
  pi/1 -> Subtract5/3
  Quadrant 6/1 -> Math Function2/2
  Subtract5/1 -> Math Function2/1  "aTrafficRel"
  Cartesian to Polar/2 -> Subtract5/1
  Selector5/1 -> Cartesian to Polar/1
  Selector1/1 -> Cartesian to Polar/2
  Subtract/1 -> Selector1/1, Selector5/1
  Selector2/1 -> Subtract/2, Sum of Elements/1
  Compare To Constant/1 -> RadarInvalid/1
  Sum of Elements/1 -> Compare To Constant/1
